simulink model "b1"  (R2020a)
settings: Solver=VariableStepAuto  StartTime=0.0  StopTime=10  RelTol=1e-3
settings Model: Creator=vivek vivian  LastModifiedBy=vivek vivian

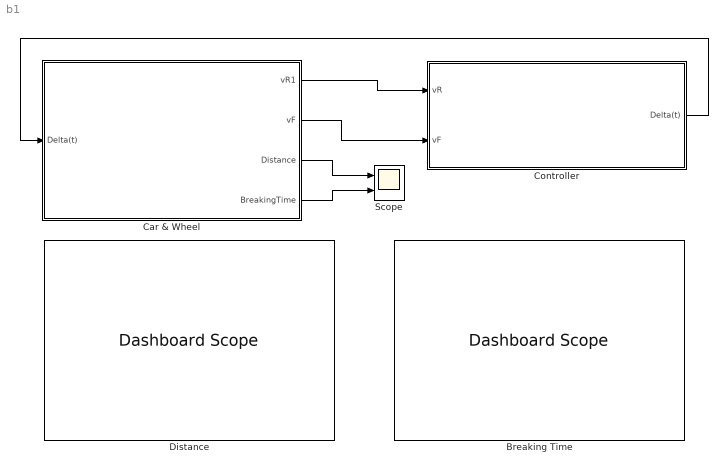
== system b1 ==
  Breaking Time : DashboardScope
  Car & Wheel : Subsystem
  Controller : Subsystem
  Distance : DashboardScope
  Scope : Scope  NumInputPorts=2
  wires:
  Controller/1(Delta(t)) -> Car & Wheel/1(Delta(t))
  Car & Wheel/1(vR1) -> Controller/1(vR)
  Car & Wheel/2(vF) -> Controller/2(vF)
  Car & Wheel/4(BreakingTime) -> Scope/2
  Car & Wheel/3(Distance) -> Scope/1

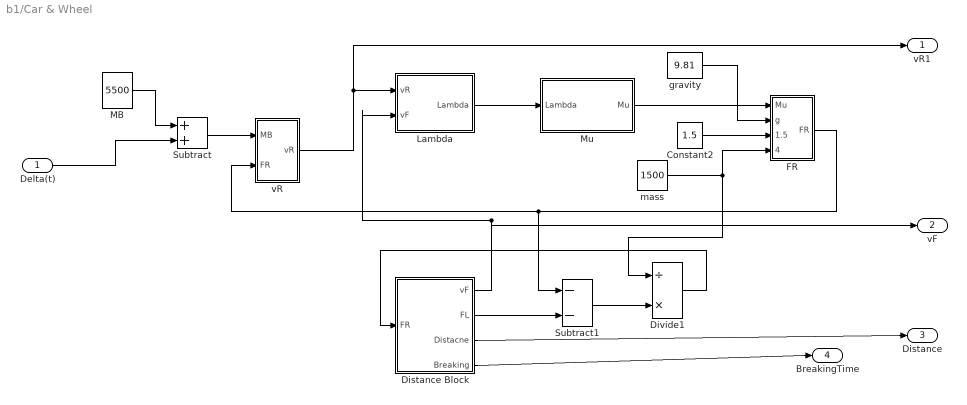
== system b1/Car & Wheel ==
  Delta(t) : Inport
  Constant2 : Constant  Value=1.5
  Distance Block : Subsystem
  Divide1 : Product  Inputs=/*
  FR : Subsystem
  Lambda : Subsystem
  MB : Constant  Value=5500
  Mu : Subsystem
  Subtract : Sum
  Subtract1 : Sum  Inputs=--
  gravity : Constant  Value=9.81
  mass : Constant  Value=1500
  vR : Subsystem
  vR1 : Outport
  vF : Outport  Port=2
  Distance : Outport  Port=3
  BreakingTime : Outport  Port=4
  wires:
  MB/1 -> Subtract/1
  gravity/1 -> FR/2(g)
  mass/1 -> FR/4(Mass), Divide1/1
  FR/1(FR) -> Subtract1/1, vR/2(FR)
  Mu/1(Mu) -> FR/1(Mu)
  Constant2/1 -> FR/3(1.5)
  Lambda/1(Lambda) -> Mu/1(Lambda)
  Distance Block/1(vF) -> Lambda/2(vF), vF/1
  Distance Block/2(FL) -> Subtract1/2
  vR/1(vR) -> vR1/1, Lambda/1(vR)
  Divide1/1 -> Distance Block/1(FR)
  Subtract/1 -> vR/1(MB)
  Subtract1/1 -> Divide1/2
  Delta(t)/1 -> Subtract/2
  Distance Block/3(Distacne) -> Distance/1
  Distance Block/4(Breaking) -> BreakingTime/1

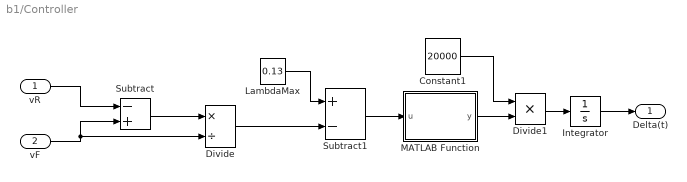
== system b1/Controller ==
  vR : Inport
  vF : Inport  Port=2
  Constant1 : Constant  Value=20000
  Divide : Product  Inputs=*/
  Divide1 : Product  Inputs=**
  Integrator : Integrator
  LambdaMax : Constant  Value=0.13
  MATLAB Function : MATLAB Function  TreatAsAtomicUnit=on
  Subtract : Sum  Inputs=-+
  Subtract1 : Sum  Inputs=+-
  Delta(t) : Outport
  wires:
  vR/1 -> Subtract/1
  vF/1 -> Subtract/2, Divide/2
  Subtract/1 -> Divide/1
  LambdaMax/1 -> Subtract1/1
  Divide/1 -> Subtract1/2
  Subtract1/1 -> MATLAB Function/1(u)
  Constant1/1 -> Divide1/1
  MATLAB Function/1(y) -> Divide1/2
  Divide1/1 -> Integrator/1
  Integrator/1 -> Delta(t)/1

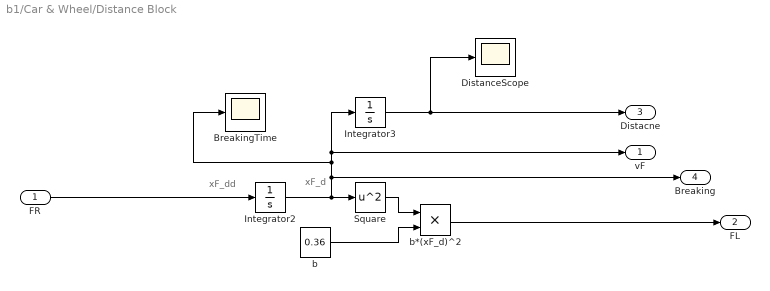
== system b1/Car & Wheel/Distance Block ==
  note: xF_dd
  note: xF_d
  FR : Inport
  BreakingTime : Scope
  DistanceScope : Scope
  Integrator2 : Integrator  InitialCondition=30  LimitOutput=on  LowerSaturationLimit=0
  Integrator3 : Integrator
  Square : Math  Operator=square  SaturateOnIntegerOverflow=on
  b : Constant  Value=0.36
  b*(xF_d)^2 : Product  Inputs=**
  vF : Outport
  FL : Outport  Port=2
  Distacne : Outport  Port=3
  Breaking : Outport  Port=4
  wires:
  Integrator2/1 -> BreakingTime/1, Integrator3/1, vF/1, Breaking/1, Square/1
  FR/1 -> Integrator2/1
  b/1 -> b*(xF_d)^2/2
  Integrator3/1 -> DistanceScope/1, Distacne/1
  Square/1 -> b*(xF_d)^2/1
  b*(xF_d)^2/1 -> FL/1

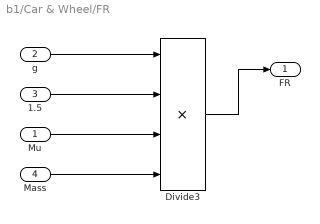
== system b1/Car & Wheel/FR ==
  Mu : Inport
  g : Inport  Port=2
  1.5 : Inport  Port=3
  Mass : Inport  Port=4
  Divide3 : Product  Inputs=****
  FR : Outport
  wires:
  1.5/1 -> Divide3/2
  g/1 -> Divide3/1
  Divide3/1 -> FR/1
  Mass/1 -> Divide3/4
  Mu/1 -> Divide3/3

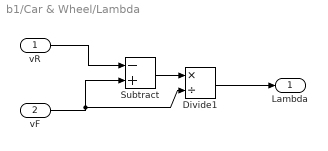
== system b1/Car & Wheel/Lambda ==
  vR : Inport
  vF : Inport  Port=2
  Divide1 : Product  Inputs=*/
  Subtract : Sum  Inputs=-+
  Lambda : Outport
  wires:
  Subtract/1 -> Divide1/1
  vF/1 -> Divide1/2, Subtract/2
  vR/1 -> Subtract/1
  Divide1/1 -> Lambda/1

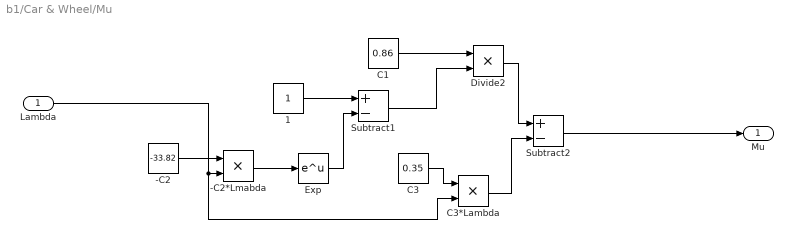
== system b1/Car & Wheel/Mu ==
  Lambda : Inport
  -C2 : Constant  Value=-33.82
  -C2*Lmabda : Product  Inputs=**
  1 : Constant
  C1 : Constant  Value=0.86
  C3 : Constant  Value=0.35
  C3*Lambda : Product  Inputs=**
  Divide2 : Product  Inputs=**
  Exp : Math  SaturateOnIntegerOverflow=on
  Subtract1 : Sum  Inputs=+-
  Subtract2 : Sum  Inputs=+-
  Mu : Outport
  wires:
  1/1 -> Subtract1/1
  -C2/1 -> -C2*Lmabda/1
  Lambda/1 -> C3*Lambda/2, -C2*Lmabda/2
  C3*Lambda/1 -> Subtract2/2
  C3/1 -> C3*Lambda/1
  -C2*Lmabda/1 -> Exp/1
  Subtract1/1 -> Divide2/2
  C1/1 -> Divide2/1
  Exp/1 -> Subtract1/2
  Divide2/1 -> Subtract2/1
  Subtract2/1 -> Mu/1

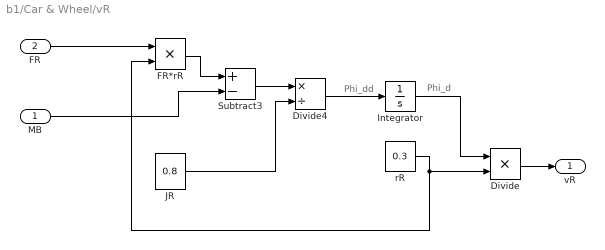
== system b1/Car & Wheel/vR ==
  note: Phi_dd
  note: Phi_d
  MB : Inport
  FR : Inport  Port=2
  Divide : Product  Inputs=**
  Divide4 : Product  Inputs=*/
  FR*rR : Product  Inputs=**
  Integrator : Integrator  InitialCondition=30  LimitOutput=on  LowerSaturationLimit=0
  JR : Constant  Value=0.8
  Subtract3 : Sum  Inputs=+-
  rR : Constant  Value=0.3
  vR : Outport
  wires:
  Divide4/1 -> Integrator/1
  rR/1 -> FR*rR/2, Divide/2
  Subtract3/1 -> Divide4/1
  Divide/1 -> vR/1
  MB/1 -> Subtract3/2
  Integrator/1 -> Divide/1
  FR/1 -> FR*rR/1
  FR*rR/1 -> Subtract3/1
  JR/1 -> Divide4/2

== matlab function b1/Controller/MATLAB Function ==
  data: u input; y output
function y = fcn(u)
if u>0
    y=1;
elseif u==0
    y = 0;
else
    y=-1;
end
